simulink model "Drone"  (R2020a)
settings: Solver=VariableStepAuto  StartTime=0.0  StopTime=t  RelTol=1e-3
values from neighbouring files (symbols this model uses):
  b = 1.84E-7    (= 1.84e-07)    [DroneControlPID.m]    (also in Drone_Control4.m = 1.98e-07; Drone_Control5.m = 1.98e-07)
  Ixx = 0.0118    [DroneControlPID.m]    (also in Drone_Control4.m = 0.0116; Drone_Control5.m = 0.0116)
  Iyy = 0.0118    [DroneControlPID.m]    (also in Drone_Control4.m = 0.0225; Drone_Control5.m = 0.0225)
  Izz = 0.0225    [DroneControlPID.m]    (also in Drone_Control4.m = 0.0121; Drone_Control5.m = 0.0121)
  k = 3.24E-8    (= 3.24e-08)    [DroneControlPID.m]    (also in Drone_Control4.m = 7.78e-06; Drone_Control5.m = 7.78e-06)
  KdPitch = KdRoll    (= 2800000)    [DroneControlPID.m]    (also in Drone_Control5.m = 841500)
  KdRoll = 2.8E6    (= 2800000)    [DroneControlPID.m]    (also in Drone_Control5.m = 1683000)
  KdYaw = 6.9E6    (= 6900000)    [DroneControlPID.m]    (also in Drone_Control5.m = 0)
  KiPitch = KiRoll    (= 3800000)    [DroneControlPID.m]    (also in Drone_Control5.m = 31684.174856)
  KiRoll = 3.8E6    (= 3800000)    [DroneControlPID.m]    (also in Drone_Control5.m = 63368.349712)
  KiYaw = 9.2E6    (= 9200000)    [DroneControlPID.m]    (also in Drone_Control5.m = 0)
  KpPitch = KpRoll    (= 6500000)    [DroneControlPID.m]    (also in Drone_Control5.m = 467500)
  KpRoll = 6.5E6    (= 6500000)    [DroneControlPID.m]    (also in Drone_Control5.m = 935000)
  KpYaw = 1.6E7    (= 16000000)    [DroneControlPID.m]    (also in Drone_Control5.m = 0)
  L = 0.225    [DroneControlPID.m]    (also in Drone_Control4.m = 160; Drone_Control5.m = 0.16)
  pitch0 = -10    [DroneControlPID.m]
  roll0 = 10    [DroneControlPID.m]
  Ts = 0.007    [DroneControlPID.m]    (also in Drone_Control5.m = 0.07)
  yaw0 = 5    [DroneControlPID.m]
libraries: simulink x3
settings Model: Creator=Evans  LastModifiedBy=Evans

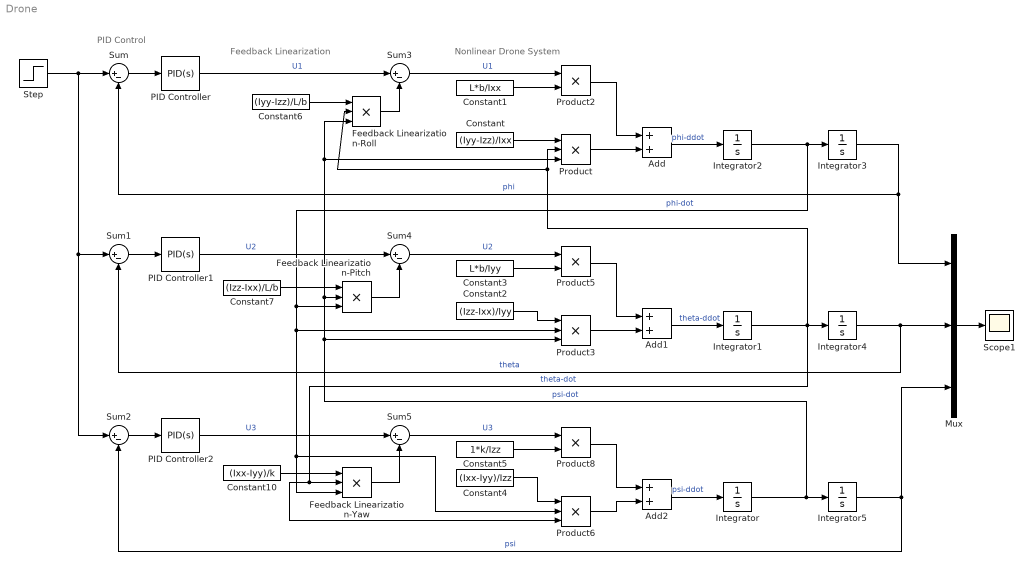
== system Drone ==
  note: Nonlinear Drone System
  note: Feedback Linearization
  note: PID Control
  Add : Sum
  Add1 : Sum
  Add2 : Sum
  Constant : Constant  Value=(Iyy-Izz)/Ixx  SampleTime=0
  Constant1 : Constant  Value=L*b/Ixx  SampleTime=0
  Constant10 : Constant  Value=(Ixx-Iyy)/k  SampleTime=0
  Constant2 : Constant  Value=(Izz-Ixx)/Iyy  SampleTime=0
  Constant3 : Constant  Value=L*b/Iyy  SampleTime=0
  Constant4 : Constant  Value=(Ixx-Iyy)/Izz  SampleTime=0
  Constant5 : Constant  Value=1*k/Izz  SampleTime=0
  Constant6 : Constant  Value=(Iyy-Izz)/L/b  SampleTime=0
  Constant7 : Constant  Value=(Izz-Ixx)/L/b  SampleTime=0
  Feedback Linearization-Pitch : Product  Inputs=3
  Feedback Linearization-Roll : Product  Inputs=3
  Feedback Linearization-Yaw : Product  Inputs=3
  Integrator : Integrator
  Integrator1 : Integrator
  Integrator2 : Integrator
  Integrator3 : Integrator  InitialCondition=deg2rad(roll0)
  Integrator4 : Integrator  InitialCondition=deg2rad(pitch0)
  Integrator5 : Integrator  InitialCondition=deg2rad(yaw0)
  Mux : Mux  Inputs=3
  PID Controller : simulink/Continuous/PID Controller  Controller=PID  Form=Parallel  TimeDomain=Continuous-time  UseExternalTs=on  SampleTime=Ts  IntegratorMethod=Forward Euler  FilterMethod=Forward Euler  ControllerParametersSource=internal  P=KpRoll  I=KiRoll  D=KdRoll  UseFilter=on  N=100  TunerSelectOption=Transfer Function Based (PID Tuner App)  InitialConditionSource=internal  InitialConditionForIntegrator=0  InitialConditionForFilter=0  DifferentiatorICPrevScaledInput=0  ExternalReset=none  TrackingMode=off  Kt=1  LimitOutput=off  UpperSaturationLimit=inf  LowerSaturationLimit=-inf  LinearizeAsGain=on  AntiWindupMode=none  Kb=1  POutMin=[]  POutMax=[]  IOutMin=[]  IOutMax=[]  DOutMin=[]  DOutMax=[]  NOutMin=[]  NOutMax=[]  SumOutMin=[]  SumOutMax=[]  SaturationOutMin=[]  SaturationOutMax=[]  PParamMin=[]  PParamMax=[]  IParamMin=[]  IParamMax=[]  DParamMin=[]  DParamMax=[]  NParamMin=[]  NParamMax=[]  KbParamMin=[]  KbParamMax=[]  KtParamMin=[]  KtParamMax=[]  KbOutMin=[]  KbOutMax=[]  KtOutMin=[]  KtOutMax=[]  IntegratorOutMin=[]  IntegratorOutMax=[]  FilterOutMin=[]  FilterOutMax=[]  SumI1OutMin=[]  SumI1OutMax=[]  SumI2OutMin=[]  SumI2OutMax=[]  SumI3OutMin=[]  SumI3OutMax=[]  SumI4OutMin=[]  SumI4OutMax=[]  SumDOutMin=[]  SumDOutMax=[]  DifferentiatorOutMin=[]  DifferentiatorOutMax=[]  FilterDiffOutCoefMin=[]  FilterDiffOutCoefMax=[]  ReciprocalOutMin=[]  ReciprocalOutMax=[]  SumDenOutMin=[]  SumDenOutMax=[]  SumNumOutMin=[]  SumNumOutMax=[]  DivideOutMin=[]  DivideOutMax=[]  UdiffTsProdOutMin=[]  UdiffTsProdOutMax=[]  NTsProdOutMin=[]  NTsProdOutMax=[]  UintegralTsProdOutMin=[]  UintegralTsProdOutMax=[]  UngainTsProdOutMin=[]  UngainTsProdOutMax=[]  IntegratorContinuousStateAttributes=''  IntegratorStateMustResolveToSignalObject=off  IntegratorRTWStateStorageClass=Auto  FilterContinuousStateAttributes=''  FilterStateMustResolveToSignalObject=off  FilterRTWStateStorageClass=Auto  ParallelPVariant=InternalParameters  IdealPVariant=Disabled  IVariant=InternalParameters  DVariant=InternalParameters  IntegratorVariant=Continuous  SatVariant=Disabled  AWVariant=Passthrough  PCopyVariant=Disabled  TRVariant=Disabled  FdbkBlocksVariant=Forward  IdealPFdbkVariant=Disabled  SatFdbkVariant=Disabled  DerivativeFilterVariant=ContFilter  NVariant=InternalParameters  NCopyVariant=Disabled  FilterICVariant=InternalICsFilter  IntegratorICVariant=InternalICs  ExternalResetVariant=Disabled  TRSumVariant=Passthrough  SumFdbkVariant=Disabled  SumVariant=Sum_PID  TsampFilterVariant=InternalTs  TsampNgainVariant=Passthrough  TsampIntegralVariant=Passthrough
  PID Controller1 : simulink/Continuous/PID Controller  Controller=PID  Form=Parallel  TimeDomain=Continuous-time  UseExternalTs=off  SampleTime=Ts  IntegratorMethod=Forward Euler  FilterMethod=Forward Euler  ControllerParametersSource=internal  P=KpPitch  I=KiPitch  D=KdPitch  UseFilter=on  N=100  TunerSelectOption=Transfer Function Based (PID Tuner App)  InitialConditionSource=internal  InitialConditionForIntegrator=0  InitialConditionForFilter=0  DifferentiatorICPrevScaledInput=0  ExternalReset=none  TrackingMode=off  Kt=1  LimitOutput=off  UpperSaturationLimit=inf  LowerSaturationLimit=-inf  LinearizeAsGain=on  AntiWindupMode=none  Kb=1  POutMin=[]  POutMax=[]  IOutMin=[]  IOutMax=[]  DOutMin=[]  DOutMax=[]  NOutMin=[]  NOutMax=[]  SumOutMin=[]  SumOutMax=[]  SaturationOutMin=[]  SaturationOutMax=[]  PParamMin=[]  PParamMax=[]  IParamMin=[]  IParamMax=[]  DParamMin=[]  DParamMax=[]  NParamMin=[]  NParamMax=[]  KbParamMin=[]  KbParamMax=[]  KtParamMin=[]  KtParamMax=[]  KbOutMin=[]  KbOutMax=[]  KtOutMin=[]  KtOutMax=[]  IntegratorOutMin=[]  IntegratorOutMax=[]  FilterOutMin=[]  FilterOutMax=[]  SumI1OutMin=[]  SumI1OutMax=[]  SumI2OutMin=[]  SumI2OutMax=[]  SumI3OutMin=[]  SumI3OutMax=[]  SumI4OutMin=[]  SumI4OutMax=[]  SumDOutMin=[]  SumDOutMax=[]  DifferentiatorOutMin=[]  DifferentiatorOutMax=[]  FilterDiffOutCoefMin=[]  FilterDiffOutCoefMax=[]  ReciprocalOutMin=[]  ReciprocalOutMax=[]  SumDenOutMin=[]  SumDenOutMax=[]  SumNumOutMin=[]  SumNumOutMax=[]  DivideOutMin=[]  DivideOutMax=[]  UdiffTsProdOutMin=[]  UdiffTsProdOutMax=[]  NTsProdOutMin=[]  NTsProdOutMax=[]  UintegralTsProdOutMin=[]  UintegralTsProdOutMax=[]  UngainTsProdOutMin=[]  UngainTsProdOutMax=[]  IntegratorContinuousStateAttributes=''  IntegratorStateMustResolveToSignalObject=off  IntegratorRTWStateStorageClass=Auto  FilterContinuousStateAttributes=''  FilterStateMustResolveToSignalObject=off  FilterRTWStateStorageClass=Auto  ParallelPVariant=InternalParameters  IdealPVariant=Disabled  IVariant=InternalParameters  DVariant=InternalParameters  IntegratorVariant=Continuous  SatVariant=Disabled  AWVariant=Passthrough  PCopyVariant=Disabled  TRVariant=Disabled  FdbkBlocksVariant=Forward  IdealPFdbkVariant=Disabled  SatFdbkVariant=Disabled  DerivativeFilterVariant=ContFilter  NVariant=InternalParameters  NCopyVariant=Disabled  FilterICVariant=InternalICsFilter  IntegratorICVariant=InternalICs  ExternalResetVariant=Disabled  TRSumVariant=Passthrough  SumFdbkVariant=Disabled  SumVariant=Sum_PID  TsampFilterVariant=InternalTs  TsampNgainVariant=Passthrough  TsampIntegralVariant=Passthrough
  PID Controller2 : simulink/Continuous/PID Controller  Controller=PID  Form=Parallel  TimeDomain=Continuous-time  UseExternalTs=off  SampleTime=Ts  IntegratorMethod=Forward Euler  FilterMethod=Forward Euler  ControllerParametersSource=internal  P=KpYaw  I=KiYaw  D=KdYaw  UseFilter=on  N=100  TunerSelectOption=Transfer Function Based (PID Tuner App)  InitialConditionSource=internal  InitialConditionForIntegrator=0  InitialConditionForFilter=0  DifferentiatorICPrevScaledInput=0  ExternalReset=none  TrackingMode=off  Kt=1  LimitOutput=off  UpperSaturationLimit=inf  LowerSaturationLimit=-inf  LinearizeAsGain=on  AntiWindupMode=none  Kb=1  POutMin=[]  POutMax=[]  IOutMin=[]  IOutMax=[]  DOutMin=[]  DOutMax=[]  NOutMin=[]  NOutMax=[]  SumOutMin=[]  SumOutMax=[]  SaturationOutMin=[]  SaturationOutMax=[]  PParamMin=[]  PParamMax=[]  IParamMin=[]  IParamMax=[]  DParamMin=[]  DParamMax=[]  NParamMin=[]  NParamMax=[]  KbParamMin=[]  KbParamMax=[]  KtParamMin=[]  KtParamMax=[]  KbOutMin=[]  KbOutMax=[]  KtOutMin=[]  KtOutMax=[]  IntegratorOutMin=[]  IntegratorOutMax=[]  FilterOutMin=[]  FilterOutMax=[]  SumI1OutMin=[]  SumI1OutMax=[]  SumI2OutMin=[]  SumI2OutMax=[]  SumI3OutMin=[]  SumI3OutMax=[]  SumI4OutMin=[]  SumI4OutMax=[]  SumDOutMin=[]  SumDOutMax=[]  DifferentiatorOutMin=[]  DifferentiatorOutMax=[]  FilterDiffOutCoefMin=[]  FilterDiffOutCoefMax=[]  ReciprocalOutMin=[]  ReciprocalOutMax=[]  SumDenOutMin=[]  SumDenOutMax=[]  SumNumOutMin=[]  SumNumOutMax=[]  DivideOutMin=[]  DivideOutMax=[]  UdiffTsProdOutMin=[]  UdiffTsProdOutMax=[]  NTsProdOutMin=[]  NTsProdOutMax=[]  UintegralTsProdOutMin=[]  UintegralTsProdOutMax=[]  UngainTsProdOutMin=[]  UngainTsProdOutMax=[]  IntegratorContinuousStateAttributes=''  IntegratorStateMustResolveToSignalObject=off  IntegratorRTWStateStorageClass=Auto  FilterContinuousStateAttributes=''  FilterStateMustResolveToSignalObject=off  FilterRTWStateStorageClass=Auto  ParallelPVariant=InternalParameters  IdealPVariant=Disabled  IVariant=InternalParameters  DVariant=InternalParameters  IntegratorVariant=Continuous  SatVariant=Disabled  AWVariant=Passthrough  PCopyVariant=Disabled  TRVariant=Disabled  FdbkBlocksVariant=Forward  IdealPFdbkVariant=Disabled  SatFdbkVariant=Disabled  DerivativeFilterVariant=ContFilter  NVariant=InternalParameters  NCopyVariant=Disabled  FilterICVariant=InternalICsFilter  IntegratorICVariant=InternalICs  ExternalResetVariant=Disabled  TRSumVariant=Passthrough  SumFdbkVariant=Disabled  SumVariant=Sum_PID  TsampFilterVariant=InternalTs  TsampNgainVariant=Passthrough  TsampIntegralVariant=Passthrough
  Product : Product  Inputs=3
  Product2 : Product
  Product3 : Product  Inputs=3
  Product5 : Product
  Product6 : Product  Inputs=3
  Product8 : Product
  Scope1 : Scope
  Step : Step  Time=0  After=0  SampleTime=0
  Sum{,1..5} (6 alike) : Sum  Inputs=|+-
  wires:
  Constant/1 -> Product/1
  Integrator1/1 -> Product6/3, Feedback Linearization-Yaw/2, Feedback Linearization-Roll/2, Product/2, Integrator4/1  "theta-dot"
  Constant1/1 -> Product2/2
  Product/1 -> Add/2
  Product2/1 -> Add/1
  Product5/1 -> Add1/1
  Constant2/1 -> Product3/1
  Product3/1 -> Add1/2
  Constant3/1 -> Product5/2
  Product8/1 -> Add2/1
  Constant4/1 -> Product6/1
  Product6/1 -> Add2/2
  Constant5/1 -> Product8/2
  Integrator2/1 -> Integrator3/1, Feedback Linearization-Yaw/3, Product6/2, Product3/2, Feedback Linearization-Pitch/3  "phi-dot"
  Add2/1 -> Integrator/1  "psi-ddot"
  Add1/1 -> Integrator1/1  "theta-ddot"
  Add/1 -> Integrator2/1  "phi-ddot"
  Integrator/1 -> Integrator5/1, Feedback Linearization-Pitch/2, Feedback Linearization-Roll/3, Product/3, Product3/3  "psi-dot"
  Integrator5/1 -> Sum2/2, Mux/3  "psi"
  Integrator4/1 -> Sum1/2, Mux/2  "theta"
  Integrator3/1 -> Sum/2, Mux/1  "phi"
  Sum/1 -> PID Controller/1
  Sum3/1 -> Product2/1  "U1"
  Sum1/1 -> PID Controller1/1
  Sum4/1 -> Product5/1  "U2"
  Sum2/1 -> PID Controller2/1
  Sum5/1 -> Product8/1  "U3"
  Mux/1 -> Scope1/1
  Step/1 -> Sum2/1, Sum1/1, Sum/1
  PID Controller/1 -> Sum3/1  "U1"
  Constant6/1 -> Feedback Linearization-Roll/1
  Feedback Linearization-Roll/1 -> Sum3/2
  Constant7/1 -> Feedback Linearization-Pitch/1
  PID Controller1/1 -> Sum4/1  "U2"
  Feedback Linearization-Pitch/1 -> Sum4/2
  PID Controller2/1 -> Sum5/1  "U3"
  Constant10/1 -> Feedback Linearization-Yaw/1
  Feedback Linearization-Yaw/1 -> Sum5/2
